simulink model "saved3"  (R2018b)
settings: Solver=VariableStepAuto  StartTime=0.0  StopTime=10.0  RelTol=1e-3
libraries: simulink x95, powerlib x8, powerlib_meascontrol x2
(part 3 of 6)

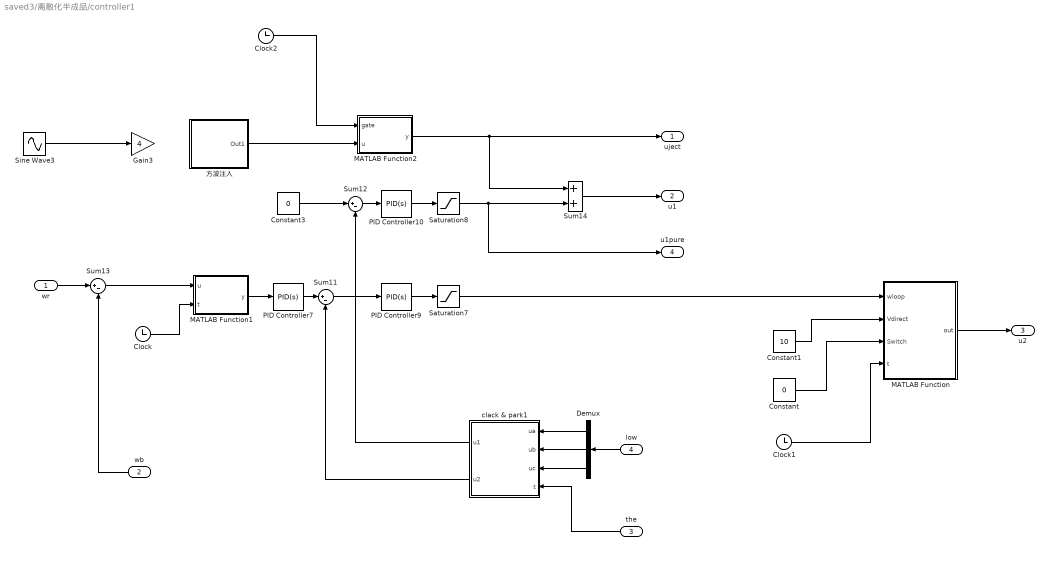
== system saved3/离散化半成品/controller1 ==
  wr : Inport
  wb : Inport  Port=2
  the : Inport  Port=3
  low : Inport  Port=4
  Clock : Clock
  Clock1 : Clock
  Clock2 : Clock
  Constant : Constant  Value=0
  Constant1 : Constant  Value=10
  Constant3 : Constant  Value=0
  Demux : Demux  Outputs=3
  Gain3 : Gain  Gain=4
  MATLAB Function : MATLAB Function  TreatAsAtomicUnit=on
  MATLAB Function1 : MATLAB Function  TreatAsAtomicUnit=on
  MATLAB Function2 : MATLAB Function  TreatAsAtomicUnit=on
  PID Controller10 : simulink/Continuous/PID Controller  Controller=PID  Form=Parallel  TimeDomain=Continuous-time  SampleTime=-1  IntegratorMethod=Forward Euler  FilterMethod=Forward Euler  ControllerParametersSource=internal  P=3  I=10  D=0  UseFilter=on  N=100  TunerSelectOption=Transfer Function Based (PID Tuner App)  InitialConditionSource=internal  InitialConditionForIntegrator=0  InitialConditionForFilter=0  DifferentiatorICPrevScaledInput=0  ExternalReset=none  TrackingMode=off  Kt=1  LimitOutput=off  UpperSaturationLimit=inf  LowerSaturationLimit=-inf  LinearizeAsGain=on  AntiWindupMode=none  Kb=1  POutMin=[]  POutMax=[]  IOutMin=[]  IOutMax=[]  DOutMin=[]  DOutMax=[]  NOutMin=[]  NOutMax=[]  SumOutMin=[]  SumOutMax=[]  SaturationOutMin=[]  SaturationOutMax=[]  PParamMin=[]  PParamMax=[]  IParamMin=[]  IParamMax=[]  DParamMin=[]  DParamMax=[]  NParamMin=[]  NParamMax=[]  KbParamMin=[]  KbParamMax=[]  KtParamMin=[]  KtParamMax=[]  KbOutMin=[]  KbOutMax=[]  KtOutMin=[]  KtOutMax=[]  IntegratorOutMin=[]  IntegratorOutMax=[]  FilterOutMin=[]  FilterOutMax=[]  SumI1OutMin=[]  SumI1OutMax=[]  SumI2OutMin=[]  SumI2OutMax=[]  SumI3OutMin=[]  SumI3OutMax=[]  SumI4OutMin=[]  SumI4OutMax=[]  SumDOutMin=[]  SumDOutMax=[]  DifferentiatorOutMin=[]  DifferentiatorOutMax=[]  FilterDiffOutCoefMin=[]  FilterDiffOutCoefMax=[]  ReciprocalOutMin=[]  ReciprocalOutMax=[]  SumDenOutMin=[]  SumDenOutMax=[]  SumNumOutMin=[]  SumNumOutMax=[]  DivideOutMin=[]  DivideOutMax=[]  IntegratorContinuousStateAttributes=''  IntegratorStateMustResolveToSignalObject=off  IntegratorRTWStateStorageClass=Auto  FilterContinuousStateAttributes=''  FilterStateMustResolveToSignalObject=off  FilterRTWStateStorageClass=Auto  ParallelPVariant=InternalParameters  IdealPVariant=Disabled  IVariant=InternalParameters  DVariant=InternalParameters  IntegratorVariant=Continuous  SatVariant=Disabled  AWVariant=Passthrough  PCopyVariant=Disabled  TRVariant=Disabled  FdbkBlocksVariant=Forward  IdealPFdbkVariant=Disabled  SatFdbkVariant=Disabled  DerivativeFilterVariant=ContFilter  NVariant=InternalParameters  NCopyVariant=Disabled  FilterICVariant=InternalICsFilter  IntegratorICVariant=InternalICs  ExternalResetVariant=Disabled  TRSumVariant=Passthrough  SumFdbkVariant=Disabled  SumVariant=Sum_PID
  PID Controller7 : simulink/Continuous/PID Controller  Controller=PID  Form=Parallel  TimeDomain=Continuous-time  SampleTime=1e-4  IntegratorMethod=Forward Euler  FilterMethod=Forward Euler  ControllerParametersSource=internal  P=0.3  I=5  D=0  UseFilter=on  N=100  TunerSelectOption=Transfer Function Based (PID Tuner App)  InitialConditionSource=internal  InitialConditionForIntegrator=0  InitialConditionForFilter=0  DifferentiatorICPrevScaledInput=0  ExternalReset=none  TrackingMode=off  Kt=1  LimitOutput=off  UpperSaturationLimit=inf  LowerSaturationLimit=-inf  LinearizeAsGain=on  AntiWindupMode=none  Kb=1  POutMin=[]  POutMax=[]  IOutMin=[]  IOutMax=[]  DOutMin=[]  DOutMax=[]  NOutMin=[]  NOutMax=[]  SumOutMin=[]  SumOutMax=[]  SaturationOutMin=[]  SaturationOutMax=[]  PParamMin=[]  PParamMax=[]  IParamMin=[]  IParamMax=[]  DParamMin=[]  DParamMax=[]  NParamMin=[]  NParamMax=[]  KbParamMin=[]  KbParamMax=[]  KtParamMin=[]  KtParamMax=[]  KbOutMin=[]  KbOutMax=[]  KtOutMin=[]  KtOutMax=[]  IntegratorOutMin=[]  IntegratorOutMax=[]  FilterOutMin=[]  FilterOutMax=[]  SumI1OutMin=[]  SumI1OutMax=[]  SumI2OutMin=[]  SumI2OutMax=[]  SumI3OutMin=[]  SumI3OutMax=[]  SumI4OutMin=[]  SumI4OutMax=[]  SumDOutMin=[]  SumDOutMax=[]  DifferentiatorOutMin=[]  DifferentiatorOutMax=[]  FilterDiffOutCoefMin=[]  FilterDiffOutCoefMax=[]  ReciprocalOutMin=[]  ReciprocalOutMax=[]  SumDenOutMin=[]  SumDenOutMax=[]  SumNumOutMin=[]  SumNumOutMax=[]  DivideOutMin=[]  DivideOutMax=[]  IntegratorContinuousStateAttributes=''  IntegratorStateMustResolveToSignalObject=off  IntegratorRTWStateStorageClass=Auto  FilterContinuousStateAttributes=''  FilterStateMustResolveToSignalObject=off  FilterRTWStateStorageClass=Auto  ParallelPVariant=InternalParameters  IdealPVariant=Disabled  IVariant=InternalParameters  DVariant=InternalParameters  IntegratorVariant=Continuous  SatVariant=Disabled  AWVariant=Passthrough  PCopyVariant=Disabled  TRVariant=Disabled  FdbkBlocksVariant=Forward  IdealPFdbkVariant=Disabled  SatFdbkVariant=Disabled  DerivativeFilterVariant=ContFilter  NVariant=InternalParameters  NCopyVariant=Disabled  FilterICVariant=InternalICsFilter  IntegratorICVariant=InternalICs  ExternalResetVariant=Disabled  TRSumVariant=Passthrough  SumFdbkVariant=Disabled  SumVariant=Sum_PID
  PID Controller9 : simulink/Continuous/PID Controller  Controller=PID  Form=Parallel  TimeDomain=Continuous-time  SampleTime=-1  IntegratorMethod=Forward Euler  FilterMethod=Forward Euler  ControllerParametersSource=internal  P=3  I=10  D=0  UseFilter=on  N=100  TunerSelectOption=Transfer Function Based (PID Tuner App)  InitialConditionSource=internal  InitialConditionForIntegrator=0  InitialConditionForFilter=0  DifferentiatorICPrevScaledInput=0  ExternalReset=none  TrackingMode=off  Kt=1  LimitOutput=off  UpperSaturationLimit=inf  LowerSaturationLimit=-inf  LinearizeAsGain=on  AntiWindupMode=none  Kb=1  POutMin=[]  POutMax=[]  IOutMin=[]  IOutMax=[]  DOutMin=[]  DOutMax=[]  NOutMin=[]  NOutMax=[]  SumOutMin=[]  SumOutMax=[]  SaturationOutMin=[]  SaturationOutMax=[]  PParamMin=[]  PParamMax=[]  IParamMin=[]  IParamMax=[]  DParamMin=[]  DParamMax=[]  NParamMin=[]  NParamMax=[]  KbParamMin=[]  KbParamMax=[]  KtParamMin=[]  KtParamMax=[]  KbOutMin=[]  KbOutMax=[]  KtOutMin=[]  KtOutMax=[]  IntegratorOutMin=[]  IntegratorOutMax=[]  FilterOutMin=[]  FilterOutMax=[]  SumI1OutMin=[]  SumI1OutMax=[]  SumI2OutMin=[]  SumI2OutMax=[]  SumI3OutMin=[]  SumI3OutMax=[]  SumI4OutMin=[]  SumI4OutMax=[]  SumDOutMin=[]  SumDOutMax=[]  DifferentiatorOutMin=[]  DifferentiatorOutMax=[]  FilterDiffOutCoefMin=[]  FilterDiffOutCoefMax=[]  ReciprocalOutMin=[]  ReciprocalOutMax=[]  SumDenOutMin=[]  SumDenOutMax=[]  SumNumOutMin=[]  SumNumOutMax=[]  DivideOutMin=[]  DivideOutMax=[]  IntegratorContinuousStateAttributes=''  IntegratorStateMustResolveToSignalObject=off  IntegratorRTWStateStorageClass=Auto  FilterContinuousStateAttributes=''  FilterStateMustResolveToSignalObject=off  FilterRTWStateStorageClass=Auto  ParallelPVariant=InternalParameters  IdealPVariant=Disabled  IVariant=InternalParameters  DVariant=InternalParameters  IntegratorVariant=Continuous  SatVariant=Disabled  AWVariant=Passthrough  PCopyVariant=Disabled  TRVariant=Disabled  FdbkBlocksVariant=Forward  IdealPFdbkVariant=Disabled  SatFdbkVariant=Disabled  DerivativeFilterVariant=ContFilter  NVariant=InternalParameters  NCopyVariant=Disabled  FilterICVariant=InternalICsFilter  IntegratorICVariant=InternalICs  ExternalResetVariant=Disabled  TRSumVariant=Passthrough  SumFdbkVariant=Disabled  SumVariant=Sum_PID
  Saturation7 : Saturate  UpperLimit=20  LowerLimit=-20
  Saturation8 : Saturate  UpperLimit=20  LowerLimit=-20
  Sine Wave3 : Sin  Frequency=1000*2*pi  SampleTime=0
  Sum11 : Sum  Inputs=|+-
  Sum12 : Sum  Inputs=|+-
  Sum13 : Sum  Inputs=|+-
  Sum14 : Sum
  clack & park1 : MATLAB Function  TreatAsAtomicUnit=on
  方波注入 : Subsystem
  uject : Outport
  u1 : Outport  Port=2
  u2 : Outport  Port=3
  u1pure : Outport  Port=4
  wires:
  Sum11/1 -> PID Controller9/1
  wb/1 -> Sum13/2
  Clock/1 -> MATLAB Function1/2(t)
  Saturation8/1 -> u1pure/1, Sum14/2
  MATLAB Function1/1(y) -> PID Controller7/1
  Sum13/1 -> MATLAB Function1/1(u)
  Constant3/1 -> Sum12/1
  PID Controller9/1 -> Saturation7/1
  Sum14/1 -> u1/1
  方波注入/1(Out1) -> MATLAB Function2/2(u)
  PID Controller7/1 -> Sum11/1
  Sum12/1 -> PID Controller10/1
  PID Controller10/1 -> Saturation8/1
  Sine Wave3/1 -> Gain3/1
  Saturation7/1 -> MATLAB Function/1(wloop)
  wr/1 -> Sum13/1
  MATLAB Function/1(out) -> u2/1
  Clock1/1 -> MATLAB Function/4(t)
  Constant/1 -> MATLAB Function/3(Switch)
  Constant1/1 -> MATLAB Function/2(Vdirect)
  Demux/1 -> clack & park1/1(ua)
  Demux/2 -> clack & park1/2(ub)
  Demux/3 -> clack & park1/3(uc)
  clack & park1/1(u1) -> Sum12/2
  clack & park1/2(u2) -> Sum11/2
  the/1 -> clack & park1/4(t)
  low/1 -> Demux/1
  MATLAB Function2/1(y) -> Sum14/1, uject/1
  Clock2/1 -> MATLAB Function2/1(gate)

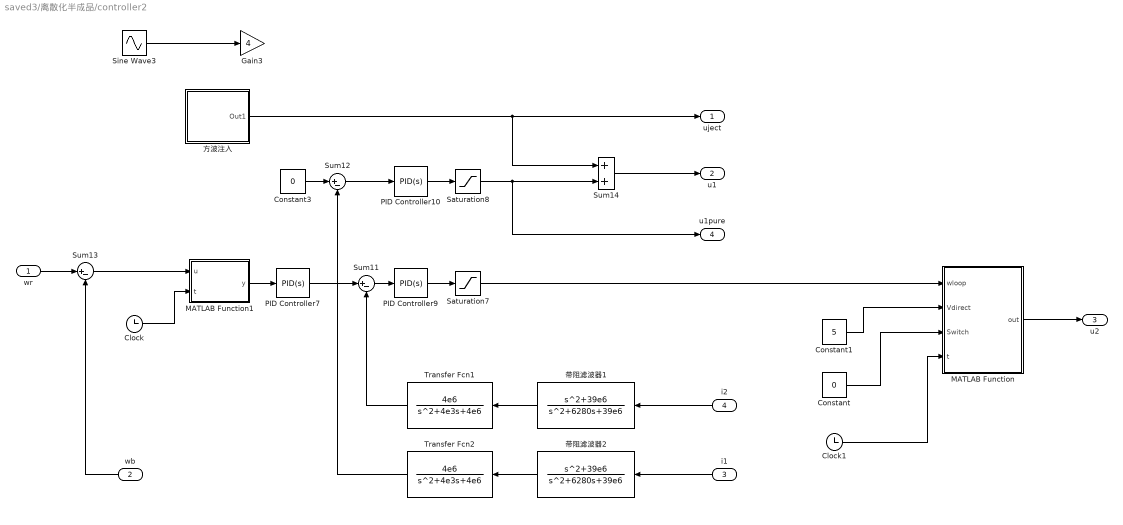
== system saved3/离散化半成品/controller2 ==
  wr : Inport
  wb : Inport  Port=2
  i1 : Inport  Port=3
  i2 : Inport  Port=4
  Clock : Clock
  Clock1 : Clock
  Constant : Constant  Value=0
  Constant1 : Constant  Value=5
  Constant3 : Constant  Value=0
  Gain3 : Gain  Gain=4
  MATLAB Function : MATLAB Function  TreatAsAtomicUnit=on
  MATLAB Function1 : MATLAB Function  TreatAsAtomicUnit=on
  PID Controller10 : simulink/Continuous/PID Controller  Controller=PID  Form=Parallel  TimeDomain=Continuous-time  SampleTime=-1  IntegratorMethod=Forward Euler  FilterMethod=Forward Euler  ControllerParametersSource=internal  P=3  I=10  D=0  UseFilter=on  N=100  TunerSelectOption=Transfer Function Based (PID Tuner App)  InitialConditionSource=internal  InitialConditionForIntegrator=0  InitialConditionForFilter=0  DifferentiatorICPrevScaledInput=0  ExternalReset=none  TrackingMode=off  Kt=1  LimitOutput=off  UpperSaturationLimit=inf  LowerSaturationLimit=-inf  LinearizeAsGain=on  AntiWindupMode=none  Kb=1  POutMin=[]  POutMax=[]  IOutMin=[]  IOutMax=[]  DOutMin=[]  DOutMax=[]  NOutMin=[]  NOutMax=[]  SumOutMin=[]  SumOutMax=[]  SaturationOutMin=[]  SaturationOutMax=[]  PParamMin=[]  PParamMax=[]  IParamMin=[]  IParamMax=[]  DParamMin=[]  DParamMax=[]  NParamMin=[]  NParamMax=[]  KbParamMin=[]  KbParamMax=[]  KtParamMin=[]  KtParamMax=[]  KbOutMin=[]  KbOutMax=[]  KtOutMin=[]  KtOutMax=[]  IntegratorOutMin=[]  IntegratorOutMax=[]  FilterOutMin=[]  FilterOutMax=[]  SumI1OutMin=[]  SumI1OutMax=[]  SumI2OutMin=[]  SumI2OutMax=[]  SumI3OutMin=[]  SumI3OutMax=[]  SumI4OutMin=[]  SumI4OutMax=[]  SumDOutMin=[]  SumDOutMax=[]  DifferentiatorOutMin=[]  DifferentiatorOutMax=[]  FilterDiffOutCoefMin=[]  FilterDiffOutCoefMax=[]  ReciprocalOutMin=[]  ReciprocalOutMax=[]  SumDenOutMin=[]  SumDenOutMax=[]  SumNumOutMin=[]  SumNumOutMax=[]  DivideOutMin=[]  DivideOutMax=[]  IntegratorContinuousStateAttributes=''  IntegratorStateMustResolveToSignalObject=off  IntegratorRTWStateStorageClass=Auto  FilterContinuousStateAttributes=''  FilterStateMustResolveToSignalObject=off  FilterRTWStateStorageClass=Auto  ParallelPVariant=InternalParameters  IdealPVariant=Disabled  IVariant=InternalParameters  DVariant=InternalParameters  IntegratorVariant=Continuous  SatVariant=Disabled  AWVariant=Passthrough  PCopyVariant=Disabled  TRVariant=Disabled  FdbkBlocksVariant=Forward  IdealPFdbkVariant=Disabled  SatFdbkVariant=Disabled  DerivativeFilterVariant=ContFilter  NVariant=InternalParameters  NCopyVariant=Disabled  FilterICVariant=InternalICsFilter  IntegratorICVariant=InternalICs  ExternalResetVariant=Disabled  TRSumVariant=Passthrough  SumFdbkVariant=Disabled  SumVariant=Sum_PID
  PID Controller7 : simulink/Continuous/PID Controller  Controller=PID  Form=Parallel  TimeDomain=Continuous-time  SampleTime=1e-4  IntegratorMethod=Forward Euler  FilterMethod=Forward Euler  ControllerParametersSource=internal  P=0.3  I=5  D=0  UseFilter=on  N=100  TunerSelectOption=Transfer Function Based (PID Tuner App)  InitialConditionSource=internal  InitialConditionForIntegrator=0  InitialConditionForFilter=0  DifferentiatorICPrevScaledInput=0  ExternalReset=none  TrackingMode=off  Kt=1  LimitOutput=off  UpperSaturationLimit=inf  LowerSaturationLimit=-inf  LinearizeAsGain=on  AntiWindupMode=none  Kb=1  POutMin=[]  POutMax=[]  IOutMin=[]  IOutMax=[]  DOutMin=[]  DOutMax=[]  NOutMin=[]  NOutMax=[]  SumOutMin=[]  SumOutMax=[]  SaturationOutMin=[]  SaturationOutMax=[]  PParamMin=[]  PParamMax=[]  IParamMin=[]  IParamMax=[]  DParamMin=[]  DParamMax=[]  NParamMin=[]  NParamMax=[]  KbParamMin=[]  KbParamMax=[]  KtParamMin=[]  KtParamMax=[]  KbOutMin=[]  KbOutMax=[]  KtOutMin=[]  KtOutMax=[]  IntegratorOutMin=[]  IntegratorOutMax=[]  FilterOutMin=[]  FilterOutMax=[]  SumI1OutMin=[]  SumI1OutMax=[]  SumI2OutMin=[]  SumI2OutMax=[]  SumI3OutMin=[]  SumI3OutMax=[]  SumI4OutMin=[]  SumI4OutMax=[]  SumDOutMin=[]  SumDOutMax=[]  DifferentiatorOutMin=[]  DifferentiatorOutMax=[]  FilterDiffOutCoefMin=[]  FilterDiffOutCoefMax=[]  ReciprocalOutMin=[]  ReciprocalOutMax=[]  SumDenOutMin=[]  SumDenOutMax=[]  SumNumOutMin=[]  SumNumOutMax=[]  DivideOutMin=[]  DivideOutMax=[]  IntegratorContinuousStateAttributes=''  IntegratorStateMustResolveToSignalObject=off  IntegratorRTWStateStorageClass=Auto  FilterContinuousStateAttributes=''  FilterStateMustResolveToSignalObject=off  FilterRTWStateStorageClass=Auto  ParallelPVariant=InternalParameters  IdealPVariant=Disabled  IVariant=InternalParameters  DVariant=InternalParameters  IntegratorVariant=Continuous  SatVariant=Disabled  AWVariant=Passthrough  PCopyVariant=Disabled  TRVariant=Disabled  FdbkBlocksVariant=Forward  IdealPFdbkVariant=Disabled  SatFdbkVariant=Disabled  DerivativeFilterVariant=ContFilter  NVariant=InternalParameters  NCopyVariant=Disabled  FilterICVariant=InternalICsFilter  IntegratorICVariant=InternalICs  ExternalResetVariant=Disabled  TRSumVariant=Passthrough  SumFdbkVariant=Disabled  SumVariant=Sum_PID
  PID Controller9 : simulink/Continuous/PID Controller  Controller=PID  Form=Parallel  TimeDomain=Continuous-time  SampleTime=-1  IntegratorMethod=Forward Euler  FilterMethod=Forward Euler  ControllerParametersSource=internal  P=3  I=10  D=0  UseFilter=on  N=100  TunerSelectOption=Transfer Function Based (PID Tuner App)  InitialConditionSource=internal  InitialConditionForIntegrator=0  InitialConditionForFilter=0  DifferentiatorICPrevScaledInput=0  ExternalReset=none  TrackingMode=off  Kt=1  LimitOutput=off  UpperSaturationLimit=inf  LowerSaturationLimit=-inf  LinearizeAsGain=on  AntiWindupMode=none  Kb=1  POutMin=[]  POutMax=[]  IOutMin=[]  IOutMax=[]  DOutMin=[]  DOutMax=[]  NOutMin=[]  NOutMax=[]  SumOutMin=[]  SumOutMax=[]  SaturationOutMin=[]  SaturationOutMax=[]  PParamMin=[]  PParamMax=[]  IParamMin=[]  IParamMax=[]  DParamMin=[]  DParamMax=[]  NParamMin=[]  NParamMax=[]  KbParamMin=[]  KbParamMax=[]  KtParamMin=[]  KtParamMax=[]  KbOutMin=[]  KbOutMax=[]  KtOutMin=[]  KtOutMax=[]  IntegratorOutMin=[]  IntegratorOutMax=[]  FilterOutMin=[]  FilterOutMax=[]  SumI1OutMin=[]  SumI1OutMax=[]  SumI2OutMin=[]  SumI2OutMax=[]  SumI3OutMin=[]  SumI3OutMax=[]  SumI4OutMin=[]  SumI4OutMax=[]  SumDOutMin=[]  SumDOutMax=[]  DifferentiatorOutMin=[]  DifferentiatorOutMax=[]  FilterDiffOutCoefMin=[]  FilterDiffOutCoefMax=[]  ReciprocalOutMin=[]  ReciprocalOutMax=[]  SumDenOutMin=[]  SumDenOutMax=[]  SumNumOutMin=[]  SumNumOutMax=[]  DivideOutMin=[]  DivideOutMax=[]  IntegratorContinuousStateAttributes=''  IntegratorStateMustResolveToSignalObject=off  IntegratorRTWStateStorageClass=Auto  FilterContinuousStateAttributes=''  FilterStateMustResolveToSignalObject=off  FilterRTWStateStorageClass=Auto  ParallelPVariant=InternalParameters  IdealPVariant=Disabled  IVariant=InternalParameters  DVariant=InternalParameters  IntegratorVariant=Continuous  SatVariant=Disabled  AWVariant=Passthrough  PCopyVariant=Disabled  TRVariant=Disabled  FdbkBlocksVariant=Forward  IdealPFdbkVariant=Disabled  SatFdbkVariant=Disabled  DerivativeFilterVariant=ContFilter  NVariant=InternalParameters  NCopyVariant=Disabled  FilterICVariant=InternalICsFilter  IntegratorICVariant=InternalICs  ExternalResetVariant=Disabled  TRSumVariant=Passthrough  SumFdbkVariant=Disabled  SumVariant=Sum_PID
  Saturation7 : Saturate  UpperLimit=20  LowerLimit=-20
  Saturation8 : Saturate  UpperLimit=20  LowerLimit=-20
  Sine Wave3 : Sin  Frequency=1000*2*pi  SampleTime=0
  Sum11 : Sum  Inputs=|+-
  Sum12 : Sum  Inputs=|+-
  Sum13 : Sum  Inputs=|+-
  Sum14 : Sum
  Transfer Fcn1 : TransferFcn  Numerator=[4e6]  Denominator=[1 4e3 4e6]
  Transfer Fcn2 : TransferFcn  Numerator=[4e6]  Denominator=[1 4e3 4e6]
  带阻滤波器1 : TransferFcn  Numerator=[1 0 39e6]  Denominator=[1 6280 39e6]
  带阻滤波器2 : TransferFcn  Numerator=[1 0 39e6]  Denominator=[1 6280 39e6]
  方波注入 : Subsystem
  uject : Outport
  u1 : Outport  Port=2
  u2 : Outport  Port=3
  u1pure : Outport  Port=4
  wires:
  Sum11/1 -> PID Controller9/1
  wb/1 -> Sum13/2
  Clock/1 -> MATLAB Function1/2(t)
  Saturation8/1 -> u1pure/1, Sum14/2
  MATLAB Function1/1(y) -> PID Controller7/1
  Sum13/1 -> MATLAB Function1/1(u)
  Constant3/1 -> Sum12/1
  PID Controller9/1 -> Saturation7/1
  Sum14/1 -> u1/1
  方波注入/1(Out1) -> uject/1, Sum14/1
  PID Controller7/1 -> Sum11/1
  Sum12/1 -> PID Controller10/1
  PID Controller10/1 -> Saturation8/1
  Sine Wave3/1 -> Gain3/1
  i2/1 -> 带阻滤波器1/1
  带阻滤波器2/1 -> Transfer Fcn2/1
  带阻滤波器1/1 -> Transfer Fcn1/1
  i1/1 -> 带阻滤波器2/1
  Saturation7/1 -> MATLAB Function/1(wloop)
  wr/1 -> Sum13/1
  Transfer Fcn1/1 -> Sum11/2
  Transfer Fcn2/1 -> Sum12/2
  MATLAB Function/1(out) -> u2/1
  Clock1/1 -> MATLAB Function/4(t)
  Constant/1 -> MATLAB Function/3(Switch)
  Constant1/1 -> MATLAB Function/2(Vdirect)

== system saved3/离散化半成品/controller3 ==
  wr : Inport
  wb : Inport  Port=2
  i1 : Inport  Port=3
  i2 : Inport  Port=4
  Clock : Clock
  Clock1 : Clock
  Constant : Constant
  Constant1 : Constant  Value=10
  Constant3 : Constant  Value=0
  Gain3 : Gain  Gain=4
  MATLAB Function : MATLAB Function  TreatAsAtomicUnit=on
  MATLAB Function1 : MATLAB Function  TreatAsAtomicUnit=on
  PID Controller10 : simulink/Continuous/PID Controller  Controller=PID  Form=Parallel  TimeDomain=Continuous-time  SampleTime=-1  IntegratorMethod=Forward Euler  FilterMethod=Forward Euler  ControllerParametersSource=internal  P=3  I=10  D=0  UseFilter=on  N=100  TunerSelectOption=Transfer Function Based (PID Tuner App)  InitialConditionSource=internal  InitialConditionForIntegrator=0  InitialConditionForFilter=0  DifferentiatorICPrevScaledInput=0  ExternalReset=none  TrackingMode=off  Kt=1  LimitOutput=off  UpperSaturationLimit=inf  LowerSaturationLimit=-inf  LinearizeAsGain=on  AntiWindupMode=none  Kb=1  POutMin=[]  POutMax=[]  IOutMin=[]  IOutMax=[]  DOutMin=[]  DOutMax=[]  NOutMin=[]  NOutMax=[]  SumOutMin=[]  SumOutMax=[]  SaturationOutMin=[]  SaturationOutMax=[]  PParamMin=[]  PParamMax=[]  IParamMin=[]  IParamMax=[]  DParamMin=[]  DParamMax=[]  NParamMin=[]  NParamMax=[]  KbParamMin=[]  KbParamMax=[]  KtParamMin=[]  KtParamMax=[]  KbOutMin=[]  KbOutMax=[]  KtOutMin=[]  KtOutMax=[]  IntegratorOutMin=[]  IntegratorOutMax=[]  FilterOutMin=[]  FilterOutMax=[]  SumI1OutMin=[]  SumI1OutMax=[]  SumI2OutMin=[]  SumI2OutMax=[]  SumI3OutMin=[]  SumI3OutMax=[]  SumI4OutMin=[]  SumI4OutMax=[]  SumDOutMin=[]  SumDOutMax=[]  DifferentiatorOutMin=[]  DifferentiatorOutMax=[]  FilterDiffOutCoefMin=[]  FilterDiffOutCoefMax=[]  ReciprocalOutMin=[]  ReciprocalOutMax=[]  SumDenOutMin=[]  SumDenOutMax=[]  SumNumOutMin=[]  SumNumOutMax=[]  DivideOutMin=[]  DivideOutMax=[]  IntegratorContinuousStateAttributes=''  IntegratorStateMustResolveToSignalObject=off  IntegratorRTWStateStorageClass=Auto  FilterContinuousStateAttributes=''  FilterStateMustResolveToSignalObject=off  FilterRTWStateStorageClass=Auto  ParallelPVariant=InternalParameters  IdealPVariant=Disabled  IVariant=InternalParameters  DVariant=InternalParameters  IntegratorVariant=Continuous  SatVariant=Disabled  AWVariant=Passthrough  PCopyVariant=Disabled  TRVariant=Disabled  FdbkBlocksVariant=Forward  IdealPFdbkVariant=Disabled  SatFdbkVariant=Disabled  DerivativeFilterVariant=ContFilter  NVariant=InternalParameters  NCopyVariant=Disabled  FilterICVariant=InternalICsFilter  IntegratorICVariant=InternalICs  ExternalResetVariant=Disabled  TRSumVariant=Passthrough  SumFdbkVariant=Disabled  SumVariant=Sum_PID
  PID Controller7 : simulink/Continuous/PID Controller  Controller=PID  Form=Parallel  TimeDomain=Continuous-time  SampleTime=1e-4  IntegratorMethod=Forward Euler  FilterMethod=Forward Euler  ControllerParametersSource=internal  P=0.3  I=5  D=0  UseFilter=on  N=100  TunerSelectOption=Transfer Function Based (PID Tuner App)  InitialConditionSource=internal  InitialConditionForIntegrator=0  InitialConditionForFilter=0  DifferentiatorICPrevScaledInput=0  ExternalReset=none  TrackingMode=off  Kt=1  LimitOutput=off  UpperSaturationLimit=inf  LowerSaturationLimit=-inf  LinearizeAsGain=on  AntiWindupMode=none  Kb=1  POutMin=[]  POutMax=[]  IOutMin=[]  IOutMax=[]  DOutMin=[]  DOutMax=[]  NOutMin=[]  NOutMax=[]  SumOutMin=[]  SumOutMax=[]  SaturationOutMin=[]  SaturationOutMax=[]  PParamMin=[]  PParamMax=[]  IParamMin=[]  IParamMax=[]  DParamMin=[]  DParamMax=[]  NParamMin=[]  NParamMax=[]  KbParamMin=[]  KbParamMax=[]  KtParamMin=[]  KtParamMax=[]  KbOutMin=[]  KbOutMax=[]  KtOutMin=[]  KtOutMax=[]  IntegratorOutMin=[]  IntegratorOutMax=[]  FilterOutMin=[]  FilterOutMax=[]  SumI1OutMin=[]  SumI1OutMax=[]  SumI2OutMin=[]  SumI2OutMax=[]  SumI3OutMin=[]  SumI3OutMax=[]  SumI4OutMin=[]  SumI4OutMax=[]  SumDOutMin=[]  SumDOutMax=[]  DifferentiatorOutMin=[]  DifferentiatorOutMax=[]  FilterDiffOutCoefMin=[]  FilterDiffOutCoefMax=[]  ReciprocalOutMin=[]  ReciprocalOutMax=[]  SumDenOutMin=[]  SumDenOutMax=[]  SumNumOutMin=[]  SumNumOutMax=[]  DivideOutMin=[]  DivideOutMax=[]  IntegratorContinuousStateAttributes=''  IntegratorStateMustResolveToSignalObject=off  IntegratorRTWStateStorageClass=Auto  FilterContinuousStateAttributes=''  FilterStateMustResolveToSignalObject=off  FilterRTWStateStorageClass=Auto  ParallelPVariant=InternalParameters  IdealPVariant=Disabled  IVariant=InternalParameters  DVariant=InternalParameters  IntegratorVariant=Continuous  SatVariant=Disabled  AWVariant=Passthrough  PCopyVariant=Disabled  TRVariant=Disabled  FdbkBlocksVariant=Forward  IdealPFdbkVariant=Disabled  SatFdbkVariant=Disabled  DerivativeFilterVariant=ContFilter  NVariant=InternalParameters  NCopyVariant=Disabled  FilterICVariant=InternalICsFilter  IntegratorICVariant=InternalICs  ExternalResetVariant=Disabled  TRSumVariant=Passthrough  SumFdbkVariant=Disabled  SumVariant=Sum_PID
  PID Controller9 : simulink/Continuous/PID Controller  Controller=PID  Form=Parallel  TimeDomain=Continuous-time  SampleTime=-1  IntegratorMethod=Forward Euler  FilterMethod=Forward Euler  ControllerParametersSource=internal  P=3  I=10  D=0  UseFilter=on  N=100  TunerSelectOption=Transfer Function Based (PID Tuner App)  InitialConditionSource=internal  InitialConditionForIntegrator=0  InitialConditionForFilter=0  DifferentiatorICPrevScaledInput=0  ExternalReset=none  TrackingMode=off  Kt=1  LimitOutput=off  UpperSaturationLimit=inf  LowerSaturationLimit=-inf  LinearizeAsGain=on  AntiWindupMode=none  Kb=1  POutMin=[]  POutMax=[]  IOutMin=[]  IOutMax=[]  DOutMin=[]  DOutMax=[]  NOutMin=[]  NOutMax=[]  SumOutMin=[]  SumOutMax=[]  SaturationOutMin=[]  SaturationOutMax=[]  PParamMin=[]  PParamMax=[]  IParamMin=[]  IParamMax=[]  DParamMin=[]  DParamMax=[]  NParamMin=[]  NParamMax=[]  KbParamMin=[]  KbParamMax=[]  KtParamMin=[]  KtParamMax=[]  KbOutMin=[]  KbOutMax=[]  KtOutMin=[]  KtOutMax=[]  IntegratorOutMin=[]  IntegratorOutMax=[]  FilterOutMin=[]  FilterOutMax=[]  SumI1OutMin=[]  SumI1OutMax=[]  SumI2OutMin=[]  SumI2OutMax=[]  SumI3OutMin=[]  SumI3OutMax=[]  SumI4OutMin=[]  SumI4OutMax=[]  SumDOutMin=[]  SumDOutMax=[]  DifferentiatorOutMin=[]  DifferentiatorOutMax=[]  FilterDiffOutCoefMin=[]  FilterDiffOutCoefMax=[]  ReciprocalOutMin=[]  ReciprocalOutMax=[]  SumDenOutMin=[]  SumDenOutMax=[]  SumNumOutMin=[]  SumNumOutMax=[]  DivideOutMin=[]  DivideOutMax=[]  IntegratorContinuousStateAttributes=''  IntegratorStateMustResolveToSignalObject=off  IntegratorRTWStateStorageClass=Auto  FilterContinuousStateAttributes=''  FilterStateMustResolveToSignalObject=off  FilterRTWStateStorageClass=Auto  ParallelPVariant=InternalParameters  IdealPVariant=Disabled  IVariant=InternalParameters  DVariant=InternalParameters  IntegratorVariant=Continuous  SatVariant=Disabled  AWVariant=Passthrough  PCopyVariant=Disabled  TRVariant=Disabled  FdbkBlocksVariant=Forward  IdealPFdbkVariant=Disabled  SatFdbkVariant=Disabled  DerivativeFilterVariant=ContFilter  NVariant=InternalParameters  NCopyVariant=Disabled  FilterICVariant=InternalICsFilter  IntegratorICVariant=InternalICs  ExternalResetVariant=Disabled  TRSumVariant=Passthrough  SumFdbkVariant=Disabled  SumVariant=Sum_PID
  Saturation7 : Saturate  UpperLimit=20  LowerLimit=-20
  Saturation8 : Saturate  UpperLimit=20  LowerLimit=-20
  Sine Wave3 : Sin  Frequency=1000*2*pi  SampleTime=0
  Sum11 : Sum  Inputs=|+-
  Sum12 : Sum  Inputs=|+-
  Sum13 : Sum  Inputs=|+-
  Sum14 : Sum
  Transfer Fcn1 : TransferFcn  Numerator=[4e6]  Denominator=[1 4e3 4e6]
  Transfer Fcn2 : TransferFcn  Numerator=[4e6]  Denominator=[1 4e3 4e6]
  带阻滤波器1 : TransferFcn  Numerator=[1 0 39e6]  Denominator=[1 6280 39e6]
  带阻滤波器2 : TransferFcn  Numerator=[1 0 39e6]  Denominator=[1 6280 39e6]
  方波注入 : Subsystem
  uject : Outport
  u1 : Outport  Port=2
  u2 : Outport  Port=3
  u1pure : Outport  Port=4
  wires:
  Sum11/1 -> PID Controller9/1
  wb/1 -> Sum13/2
  Clock/1 -> MATLAB Function1/2(t)
  Saturation8/1 -> u1pure/1, Sum14/2
  MATLAB Function1/1(y) -> PID Controller7/1
  Sum13/1 -> MATLAB Function1/1(u)
  Constant3/1 -> Sum12/1
  PID Controller9/1 -> Saturation7/1
  Sum14/1 -> u1/1
  方波注入/1(Out1) -> uject/1, Sum14/1
  PID Controller7/1 -> Sum11/1
  Sum12/1 -> PID Controller10/1
  PID Controller10/1 -> Saturation8/1
  Sine Wave3/1 -> Gain3/1
  i2/1 -> 带阻滤波器1/1
  带阻滤波器2/1 -> Transfer Fcn2/1
  带阻滤波器1/1 -> Transfer Fcn1/1
  i1/1 -> 带阻滤波器2/1
  Saturation7/1 -> MATLAB Function/1(wloop)
  wr/1 -> Sum13/1
  Transfer Fcn1/1 -> Sum11/2
  Transfer Fcn2/1 -> Sum12/2
  MATLAB Function/1(out) -> u2/1
  Clock1/1 -> MATLAB Function/4(t)
  Constant/1 -> MATLAB Function/3(Switch)
  Constant1/1 -> MATLAB Function/2(Vdirect)

== system saved3/离散化半成品/current seperator ==
  ia : Inport
  ib : Inport  Port=2
  ic : Inport  Port=3
  Mux : Mux  Inputs=3
  Mux1 : Mux  Inputs=3
  Transfer Fcn : TransferFcn  Numerator=[4e6]  Denominator=[1 4e3 4e6]
  Transfer Fcn1 : TransferFcn  Numerator=[6280 0]  Denominator=[1 6280 39e6]
  Transfer Fcn2 : TransferFcn  Numerator=[4e6]  Denominator=[1 4e3 4e6]
  Transfer Fcn3 : TransferFcn  Numerator=[6280 0]  Denominator=[1 6280 39e6]
  Transfer Fcn4 : TransferFcn  Numerator=[6280 0]  Denominator=[1 6280 39e6]
  Transfer Fcn5 : TransferFcn  Numerator=[4e6]  Denominator=[1 4e3 4e6]
  带通滤波器1 : TransferFcn  Numerator=[6280 0]  Denominator=[1 6280 39e6]
  带通滤波器3 : TransferFcn  Numerator=[6280 0]  Denominator=[1 6280 39e6]
  带通滤波器4 : TransferFcn  Numerator=[6280 0]  Denominator=[1 6280 39e6]
  带阻滤波器 : TransferFcn  Numerator=[1 0 39e6]  Denominator=[1 6280 39e6]
  带阻滤波器1 : TransferFcn  Numerator=[1 0 39e6]  Denominator=[1 6280 39e6]
  带阻滤波器2 : TransferFcn  Numerator=[1 0 39e6]  Denominator=[1 6280 39e6]
  电流采样 : Subsystem
  电流采样1 : Subsystem
  1000Hz : Outport
  low : Outport  Port=2
  wires:
  Mux/1 -> 1000Hz/1
  带通滤波器3/1 -> Transfer Fcn3/1
  Transfer Fcn1/1 -> 电流采样/1(<Stator current is_a (A)>)
  电流采样/2(ib) -> Mux/2
  电流采样/3(ic) -> Mux/3
  电流采样/1(ia) -> Mux/1
  Transfer Fcn3/1 -> 电流采样/2(<Stator current is_b (A)>)
  Transfer Fcn4/1 -> 电流采样/3(<Stator current is_c (A)>)
  带通滤波器1/1 -> Transfer Fcn1/1
  带通滤波器4/1 -> Transfer Fcn4/1
  ia/1 -> 带阻滤波器1/1, 带通滤波器1/1
  ib/1 -> 带阻滤波器/1, 带通滤波器3/1
  ic/1 -> 带阻滤波器2/1, 带通滤波器4/1
  带阻滤波器1/1 -> Transfer Fcn/1
  带阻滤波器/1 -> Transfer Fcn2/1
  Transfer Fcn2/1 -> 电流采样1/2(<Stator current is_b (A)>)
  Transfer Fcn/1 -> 电流采样1/1(<Stator current is_a (A)>)
  Transfer Fcn5/1 -> 电流采样1/3(<Stator current is_c (A)>)
  Mux1/1 -> low/1
  电流采样1/1(ia) -> Mux1/1
  电流采样1/2(ib) -> Mux1/2
  电流采样1/3(ic) -> Mux1/3
  带阻滤波器2/1 -> Transfer Fcn5/1

== system saved3/离散化半成品/inject estimater ==
  uject : Inport
  u2 : Inport  Port=2
  Gain6 : Gain  Gain=0.01
  Gain8 : Gain  Gain=-100
  Integrator2 : Integrator  InitialCondition=0.3
  PID Controller2 : simulink/Continuous/PID Controller  Controller=PID  Form=Parallel  TimeDomain=Continuous-time  SampleTime=-1  IntegratorMethod=Forward Euler  FilterMethod=Forward Euler  ControllerParametersSource=internal  P=4  I=350  D=0  UseFilter=on  N=100  TunerSelectOption=Transfer Function Based (PID Tuner App)  InitialConditionSource=internal  InitialConditionForIntegrator=0  InitialConditionForFilter=0  DifferentiatorICPrevScaledInput=0  ExternalReset=none  TrackingMode=off  Kt=1  LimitOutput=off  UpperSaturationLimit=inf  LowerSaturationLimit=-inf  LinearizeAsGain=on  AntiWindupMode=none  Kb=1  POutMin=[]  POutMax=[]  IOutMin=[]  IOutMax=[]  DOutMin=[]  DOutMax=[]  NOutMin=[]  NOutMax=[]  SumOutMin=[]  SumOutMax=[]  SaturationOutMin=[]  SaturationOutMax=[]  PParamMin=[]  PParamMax=[]  IParamMin=[]  IParamMax=[]  DParamMin=[]  DParamMax=[]  NParamMin=[]  NParamMax=[]  KbParamMin=[]  KbParamMax=[]  KtParamMin=[]  KtParamMax=[]  KbOutMin=[]  KbOutMax=[]  KtOutMin=[]  KtOutMax=[]  IntegratorOutMin=[]  IntegratorOutMax=[]  FilterOutMin=[]  FilterOutMax=[]  SumI1OutMin=[]  SumI1OutMax=[]  SumI2OutMin=[]  SumI2OutMax=[]  SumI3OutMin=[]  SumI3OutMax=[]  SumI4OutMin=[]  SumI4OutMax=[]  SumDOutMin=[]  SumDOutMax=[]  DifferentiatorOutMin=[]  DifferentiatorOutMax=[]  FilterDiffOutCoefMin=[]  FilterDiffOutCoefMax=[]  ReciprocalOutMin=[]  ReciprocalOutMax=[]  SumDenOutMin=[]  SumDenOutMax=[]  SumNumOutMin=[]  SumNumOutMax=[]  DivideOutMin=[]  DivideOutMax=[]  IntegratorContinuousStateAttributes=''  IntegratorStateMustResolveToSignalObject=off  IntegratorRTWStateStorageClass=Auto  FilterContinuousStateAttributes=''  FilterStateMustResolveToSignalObject=off  FilterRTWStateStorageClass=Auto  ParallelPVariant=InternalParameters  IdealPVariant=Disabled  IVariant=InternalParameters  DVariant=InternalParameters  IntegratorVariant=Continuous  SatVariant=Disabled  AWVariant=Passthrough  PCopyVariant=Disabled  TRVariant=Disabled  FdbkBlocksVariant=Forward  IdealPFdbkVariant=Disabled  SatFdbkVariant=Disabled  DerivativeFilterVariant=ContFilter  NVariant=InternalParameters  NCopyVariant=Disabled  FilterICVariant=InternalICsFilter  IntegratorICVariant=InternalICs  ExternalResetVariant=Disabled  TRSumVariant=Passthrough  SumFdbkVariant=Disabled  SumVariant=Sum_PID
  Ramp2 : simulink/Sources/Ramp  slope=0  start=0  InitialOutput=0
  Scope19 : Scope
  Scope7 : Scope  NumInputPorts=2
  Sum2 : Sum  Inputs=|++
  Transfer Fcn2 : TransferFcn  Numerator=[6280 0]  Denominator=[1 6280 39e6]
  低通滤波器 : TransferFcn  Numerator=[25e4]  Denominator=[1 500 25e4]
  带通滤波器1 : TransferFcn  Numerator=[6280 0]  Denominator=[1 6280 39e6]
  带通滤波器2 : TransferFcn  Numerator=[6280 0]  Denominator=[1 6280 39e6]
  混频 : Product
  相移器-90° : TransferFcn  Numerator=[39e6]  Denominator=[1 6280 39e6]
  theHat : Outport
  wHat : Outport  Port=2
  wires:
  相移器-90°/1 -> 混频/1
  混频/1 -> 低通滤波器/1
  Gain6/1 -> Scope7/1
  带通滤波器2/1 -> Transfer Fcn2/1
  Transfer Fcn2/1 -> 相移器-90°/1, Scope7/2
  PID Controller2/1 -> Sum2/1
  Integrator2/1 -> theHat/1
  Gain8/1 -> PID Controller2/1
  Ramp2/1 -> Sum2/2
  带通滤波器1/1 -> 混频/2, Gain6/1
  u2/1 -> 带通滤波器2/1
  uject/1 -> 带通滤波器1/1
  Sum2/1 -> wHat/1, Integrator2/1
  低通滤波器/1 -> Gain8/1, Scope19/1

== system saved3/离散化半成品/inject estimater(digital) ==
  uject : Inport
  u2 : Inport  Port=2
  Constant : Constant  Value=1000
  Constant1 : Constant  Value=0.3
  Gain1 : Gain  Gain=-3
  Gain6 : Gain  Gain=0.01
  Scope : Scope
  Scope1 : Scope  NumInputPorts=2
  Sum : Sum  Inputs=|++
  Transfer Fcn2 : TransferFcn  Numerator=[6280 0]  Denominator=[1 6280 39e6]
  乘法 : Product
  带通滤波器2 : TransferFcn  Numerator=[6280 0]  Denominator=[1 6280 39e6]
  鉴幅鉴相器(可选快速门滑窗) : MATLAB Function  TreatAsAtomicUnit=on  SystemSampleTime=1e-4
  锁相器 : MATLAB Function  TreatAsAtomicUnit=on  SystemSampleTime=1e-4
  theHat : Outport
  wHat : Outport  Port=2
  wires:
  带通滤波器2/1 -> Transfer Fcn2/1
  Transfer Fcn2/1 -> 鉴幅鉴相器(可选快速门滑窗)/2(S2), Scope1/2
  Gain1/1 -> 锁相器/1(u)
  uject/1 -> 鉴幅鉴相器(可选快速门滑窗)/1(S1), Gain6/1
  u2/1 -> 带通滤波器2/1
  鉴幅鉴相器(可选快速门滑窗)/2(A2) -> 乘法/1
  鉴幅鉴相器(可选快速门滑窗)/3(DP) -> 乘法/2  "phase"
  乘法/1 -> Gain1/1, Scope/1
  Constant/1 -> 鉴幅鉴相器(可选快速门滑窗)/3(Fre)
  Gain6/1 -> Scope1/1
  Sum/1 -> theHat/1
  Constant1/1 -> Sum/2
  锁相器/1(the) -> Sum/1
  锁相器/2(w) -> wHat/1

== system saved3/离散化半成品/inject estimater(digital)1 ==
  uject : Inport
  In3 : Inport  Port=2
  Constant2 : Constant  Value=1000
  Constant3 : Constant  Value=0.3
  Delay : Delay  DelayLength=1
  Demux : Demux  Outputs=3
  Gain2 : Gain  Gain=-3
  Gain3 : Gain  Gain=0.01
  Scope2 : Scope
  Scope3 : Scope  NumInputPorts=2
  Sum1 : Sum  Inputs=|++
  clack & park2 : MATLAB Function  TreatAsAtomicUnit=on
  乘法1 : Product
  鉴幅鉴相器(可选快速门滑窗)1 : MATLAB Function  TreatAsAtomicUnit=on  SystemSampleTime=1e-4
  锁相器1 : MATLAB Function  TreatAsAtomicUnit=on  SystemSampleTime=1e-4
  the : Outport
  wHat : Outport  Port=2
  wires:
  uject/1 -> 鉴幅鉴相器(可选快速门滑窗)1/1(S1), Gain3/1
  In3/1 -> Demux/1
  Gain2/1 -> 锁相器1/1(u)
  Constant2/1 -> 鉴幅鉴相器(可选快速门滑窗)1/3(Fre)
  鉴幅鉴相器(可选快速门滑窗)1/3(DP) -> 乘法1/2  "phase"
  鉴幅鉴相器(可选快速门滑窗)1/2(A2) -> 乘法1/1
  乘法1/1 -> Gain2/1, Scope2/1
  Gain3/1 -> Scope3/1
  Constant3/1 -> Sum1/2
  Demux/1 -> clack & park2/1(ua)
  Demux/2 -> clack & park2/2(ub)
  Demux/3 -> clack & park2/3(uc)
  锁相器1/2(w) -> wHat/1
  锁相器1/1(the) -> Sum1/1
  Sum1/1 -> Delay/1, the/1
  clack & park2/2(u2) -> 鉴幅鉴相器(可选快速门滑窗)1/2(S2), Scope3/2
  Delay/1 -> clack & park2/4(t)

== system saved3/离散化半成品/inject estimater(digital)2 ==
  uject : Inport
  In3 : Inport  Port=2
  Constant2 : Constant  Value=1000
  Constant3 : Constant  Value=0.3
  Delay : Delay  DelayLength=1
  Demux : Demux  Outputs=3
  Gain2 : Gain  Gain=-3
  Gain3 : Gain  Gain=0.01
  Scope2 : Scope
  Scope3 : Scope  NumInputPorts=2
  Sum1 : Sum  Inputs=|++
  clack & park2 : MATLAB Function  TreatAsAtomicUnit=on
  乘法1 : Product
  鉴幅鉴相器(可选快速门滑窗)1 : MATLAB Function  TreatAsAtomicUnit=on  SystemSampleTime=1e-4
  锁相器1 : MATLAB Function  TreatAsAtomicUnit=on  SystemSampleTime=1e-4
  the : Outport
  wHat : Outport  Port=2
  wires:
  uject/1 -> 鉴幅鉴相器(可选快速门滑窗)1/1(S1), Gain3/1
  In3/1 -> Demux/1
  Gain2/1 -> 锁相器1/1(u)
  Constant2/1 -> 鉴幅鉴相器(可选快速门滑窗)1/3(Fre)
  鉴幅鉴相器(可选快速门滑窗)1/3(DP) -> 乘法1/2  "phase"
  鉴幅鉴相器(可选快速门滑窗)1/2(A2) -> 乘法1/1
  乘法1/1 -> Gain2/1, Scope2/1
  Gain3/1 -> Scope3/1
  Constant3/1 -> Sum1/2
  Demux/1 -> clack & park2/1(ua)
  Demux/2 -> clack & park2/2(ub)
  Demux/3 -> clack & park2/3(uc)
  锁相器1/2(w) -> wHat/1
  锁相器1/1(the) -> Sum1/1
  Sum1/1 -> Delay/1, the/1
  clack & park2/2(u2) -> 鉴幅鉴相器(可选快速门滑窗)1/2(S2), Scope3/2
  Delay/1 -> clack & park2/4(t)

== system saved3/离散化半成品/inject estimater(digital)3 ==
  uject : Inport
  u2 : Inport  Port=2
  Constant : Constant  Value=1000
  Constant1 : Constant  Value=0.3
  Gain1 : Gain  Gain=-3
  Gain6 : Gain  Gain=0.01
  Scope : Scope
  Scope1 : Scope  NumInputPorts=2
  Sum : Sum  Inputs=|++
  Transfer Fcn2 : TransferFcn  Numerator=[6280 0]  Denominator=[1 6280 39e6]
  乘法 : Product
  带通滤波器2 : TransferFcn  Numerator=[6280 0]  Denominator=[1 6280 39e6]
  鉴幅鉴相器(可选快速门滑窗) : MATLAB Function  TreatAsAtomicUnit=on  SystemSampleTime=1e-4
  锁相器 : MATLAB Function  TreatAsAtomicUnit=on  SystemSampleTime=1e-4
  theHat : Outport
  wHat : Outport  Port=2
  wires:
  带通滤波器2/1 -> Transfer Fcn2/1
  Transfer Fcn2/1 -> 鉴幅鉴相器(可选快速门滑窗)/2(S2), Scope1/2
  Gain1/1 -> 锁相器/1(u)
  uject/1 -> 鉴幅鉴相器(可选快速门滑窗)/1(S1), Gain6/1
  u2/1 -> 带通滤波器2/1
  鉴幅鉴相器(可选快速门滑窗)/2(A2) -> 乘法/1
  鉴幅鉴相器(可选快速门滑窗)/3(DP) -> 乘法/2  "phase"
  乘法/1 -> Gain1/1, Scope/1
  Constant/1 -> 鉴幅鉴相器(可选快速门滑窗)/3(Fre)
  Gain6/1 -> Scope1/1
  Sum/1 -> theHat/1
  Constant1/1 -> Sum/2
  锁相器/1(the) -> Sum/1
  锁相器/2(w) -> wHat/1

== system saved3/离散化半成品/inject estimater1 ==
  uject : Inport
  u2 : Inport  Port=2
  Gain6 : Gain  Gain=0.01
  Gain8 : Gain  Gain=-100
  Integrator2 : Integrator  InitialCondition=0.3
  PID Controller2 : simulink/Continuous/PID Controller  Controller=PID  Form=Parallel  TimeDomain=Continuous-time  SampleTime=-1  IntegratorMethod=Forward Euler  FilterMethod=Forward Euler  ControllerParametersSource=internal  P=4  I=350  D=0  UseFilter=on  N=100  TunerSelectOption=Transfer Function Based (PID Tuner App)  InitialConditionSource=internal  InitialConditionForIntegrator=0  InitialConditionForFilter=0  DifferentiatorICPrevScaledInput=0  ExternalReset=none  TrackingMode=off  Kt=1  LimitOutput=off  UpperSaturationLimit=inf  LowerSaturationLimit=-inf  LinearizeAsGain=on  AntiWindupMode=none  Kb=1  POutMin=[]  POutMax=[]  IOutMin=[]  IOutMax=[]  DOutMin=[]  DOutMax=[]  NOutMin=[]  NOutMax=[]  SumOutMin=[]  SumOutMax=[]  SaturationOutMin=[]  SaturationOutMax=[]  PParamMin=[]  PParamMax=[]  IParamMin=[]  IParamMax=[]  DParamMin=[]  DParamMax=[]  NParamMin=[]  NParamMax=[]  KbParamMin=[]  KbParamMax=[]  KtParamMin=[]  KtParamMax=[]  KbOutMin=[]  KbOutMax=[]  KtOutMin=[]  KtOutMax=[]  IntegratorOutMin=[]  IntegratorOutMax=[]  FilterOutMin=[]  FilterOutMax=[]  SumI1OutMin=[]  SumI1OutMax=[]  SumI2OutMin=[]  SumI2OutMax=[]  SumI3OutMin=[]  SumI3OutMax=[]  SumI4OutMin=[]  SumI4OutMax=[]  SumDOutMin=[]  SumDOutMax=[]  DifferentiatorOutMin=[]  DifferentiatorOutMax=[]  FilterDiffOutCoefMin=[]  FilterDiffOutCoefMax=[]  ReciprocalOutMin=[]  ReciprocalOutMax=[]  SumDenOutMin=[]  SumDenOutMax=[]  SumNumOutMin=[]  SumNumOutMax=[]  DivideOutMin=[]  DivideOutMax=[]  IntegratorContinuousStateAttributes=''  IntegratorStateMustResolveToSignalObject=off  IntegratorRTWStateStorageClass=Auto  FilterContinuousStateAttributes=''  FilterStateMustResolveToSignalObject=off  FilterRTWStateStorageClass=Auto  ParallelPVariant=InternalParameters  IdealPVariant=Disabled  IVariant=InternalParameters  DVariant=InternalParameters  IntegratorVariant=Continuous  SatVariant=Disabled  AWVariant=Passthrough  PCopyVariant=Disabled  TRVariant=Disabled  FdbkBlocksVariant=Forward  IdealPFdbkVariant=Disabled  SatFdbkVariant=Disabled  DerivativeFilterVariant=ContFilter  NVariant=InternalParameters  NCopyVariant=Disabled  FilterICVariant=InternalICsFilter  IntegratorICVariant=InternalICs  ExternalResetVariant=Disabled  TRSumVariant=Passthrough  SumFdbkVariant=Disabled  SumVariant=Sum_PID
  Ramp2 : simulink/Sources/Ramp  slope=0  start=0  InitialOutput=0
  Scope19 : Scope
  Scope7 : Scope  NumInputPorts=2
  Sum2 : Sum  Inputs=|++
  Transfer Fcn2 : TransferFcn  Numerator=[6280 0]  Denominator=[1 6280 39e6]
  低通滤波器 : TransferFcn  Numerator=[25e4]  Denominator=[1 500 25e4]
  带通滤波器1 : TransferFcn  Numerator=[6280 0]  Denominator=[1 6280 39e6]
  带通滤波器2 : TransferFcn  Numerator=[6280 0]  Denominator=[1 6280 39e6]
  混频 : Product
  相移器-90° : TransferFcn  Numerator=[39e6]  Denominator=[1 6280 39e6]
  theHat : Outport
  wHat : Outport  Port=2
  wires:
  相移器-90°/1 -> 混频/1
  混频/1 -> 低通滤波器/1
  Gain6/1 -> Scope7/1
  带通滤波器2/1 -> Transfer Fcn2/1
  Transfer Fcn2/1 -> 相移器-90°/1, Scope7/2
  PID Controller2/1 -> Sum2/1
  Integrator2/1 -> theHat/1
  Gain8/1 -> PID Controller2/1
  Ramp2/1 -> Sum2/2
  带通滤波器1/1 -> 混频/2, Gain6/1
  u2/1 -> 带通滤波器2/1
  uject/1 -> 带通滤波器1/1
  Sum2/1 -> wHat/1, Integrator2/1
  低通滤波器/1 -> Gain8/1, Scope19/1

== system saved3/离散化半成品/inject estimater2 ==
  uject : Inport
  u2 : Inport  Port=2
  Gain6 : Gain  Gain=0.01
  Gain8 : Gain  Gain=-100
  Integrator2 : Integrator  InitialCondition=0.3
  PID Controller2 : simulink/Continuous/PID Controller  Controller=PID  Form=Parallel  TimeDomain=Continuous-time  SampleTime=-1  IntegratorMethod=Forward Euler  FilterMethod=Forward Euler  ControllerParametersSource=internal  P=4  I=350  D=0  UseFilter=on  N=100  TunerSelectOption=Transfer Function Based (PID Tuner App)  InitialConditionSource=internal  InitialConditionForIntegrator=0  InitialConditionForFilter=0  DifferentiatorICPrevScaledInput=0  ExternalReset=none  TrackingMode=off  Kt=1  LimitOutput=off  UpperSaturationLimit=inf  LowerSaturationLimit=-inf  LinearizeAsGain=on  AntiWindupMode=none  Kb=1  POutMin=[]  POutMax=[]  IOutMin=[]  IOutMax=[]  DOutMin=[]  DOutMax=[]  NOutMin=[]  NOutMax=[]  SumOutMin=[]  SumOutMax=[]  SaturationOutMin=[]  SaturationOutMax=[]  PParamMin=[]  PParamMax=[]  IParamMin=[]  IParamMax=[]  DParamMin=[]  DParamMax=[]  NParamMin=[]  NParamMax=[]  KbParamMin=[]  KbParamMax=[]  KtParamMin=[]  KtParamMax=[]  KbOutMin=[]  KbOutMax=[]  KtOutMin=[]  KtOutMax=[]  IntegratorOutMin=[]  IntegratorOutMax=[]  FilterOutMin=[]  FilterOutMax=[]  SumI1OutMin=[]  SumI1OutMax=[]  SumI2OutMin=[]  SumI2OutMax=[]  SumI3OutMin=[]  SumI3OutMax=[]  SumI4OutMin=[]  SumI4OutMax=[]  SumDOutMin=[]  SumDOutMax=[]  DifferentiatorOutMin=[]  DifferentiatorOutMax=[]  FilterDiffOutCoefMin=[]  FilterDiffOutCoefMax=[]  ReciprocalOutMin=[]  ReciprocalOutMax=[]  SumDenOutMin=[]  SumDenOutMax=[]  SumNumOutMin=[]  SumNumOutMax=[]  DivideOutMin=[]  DivideOutMax=[]  IntegratorContinuousStateAttributes=''  IntegratorStateMustResolveToSignalObject=off  IntegratorRTWStateStorageClass=Auto  FilterContinuousStateAttributes=''  FilterStateMustResolveToSignalObject=off  FilterRTWStateStorageClass=Auto  ParallelPVariant=InternalParameters  IdealPVariant=Disabled  IVariant=InternalParameters  DVariant=InternalParameters  IntegratorVariant=Continuous  SatVariant=Disabled  AWVariant=Passthrough  PCopyVariant=Disabled  TRVariant=Disabled  FdbkBlocksVariant=Forward  IdealPFdbkVariant=Disabled  SatFdbkVariant=Disabled  DerivativeFilterVariant=ContFilter  NVariant=InternalParameters  NCopyVariant=Disabled  FilterICVariant=InternalICsFilter  IntegratorICVariant=InternalICs  ExternalResetVariant=Disabled  TRSumVariant=Passthrough  SumFdbkVariant=Disabled  SumVariant=Sum_PID
  Ramp2 : simulink/Sources/Ramp  slope=0  start=0  InitialOutput=0
  Scope19 : Scope
  Scope7 : Scope  NumInputPorts=2
  Sum2 : Sum  Inputs=|++
  Transfer Fcn2 : TransferFcn  Numerator=[6280 0]  Denominator=[1 6280 39e6]
  低通滤波器 : TransferFcn  Numerator=[25e4]  Denominator=[1 500 25e4]
  带通滤波器1 : TransferFcn  Numerator=[6280 0]  Denominator=[1 6280 39e6]
  带通滤波器2 : TransferFcn  Numerator=[6280 0]  Denominator=[1 6280 39e6]
  混频 : Product
  相移器-90° : TransferFcn  Numerator=[39e6]  Denominator=[1 6280 39e6]
  theHat : Outport
  wHat : Outport  Port=2
  wires:
  相移器-90°/1 -> 混频/1
  混频/1 -> 低通滤波器/1
  Gain6/1 -> Scope7/1
  带通滤波器2/1 -> Transfer Fcn2/1
  Transfer Fcn2/1 -> 相移器-90°/1, Scope7/2
  PID Controller2/1 -> Sum2/1
  Integrator2/1 -> theHat/1
  Gain8/1 -> PID Controller2/1
  Ramp2/1 -> Sum2/2
  带通滤波器1/1 -> 混频/2, Gain6/1
  u2/1 -> 带通滤波器2/1
  uject/1 -> 带通滤波器1/1
  Sum2/1 -> wHat/1, Integrator2/1
  低通滤波器/1 -> Gain8/1, Scope19/1

== system saved3/离散化半成品/w estimater ==
  u1pure : Inport
  u2 : Inport  Port=2
  ia : Inport  Port=3
  ib : Inport  Port=4
  ic : Inport  Port=5
  the : Inport  Port=6
  MATLAB Function : MATLAB Function  TreatAsAtomicUnit=on
  Subsystem : Subsystem
  Transfer Fcn : TransferFcn  Numerator=[4e6]  Denominator=[1 4e3 4e6]
  Transfer Fcn1 : TransferFcn  Numerator=[4e6]  Denominator=[1 4e3 4e6]
  clack : MATLAB Function  TreatAsAtomicUnit=on
  iabc : Scope  NumInputPorts=3
  invpark : MATLAB Function  TreatAsAtomicUnit=on
  带阻滤波器 : TransferFcn  Numerator=[1 0 39e6]  Denominator=[1 6280 39e6]
  带阻滤波器1 : TransferFcn  Numerator=[1 0 39e6]  Denominator=[1 6280 39e6]
  锁相环 : Subsystem
  wHat : Outport
  theHat : Outport  Port=2
  wires:
  ib/1 -> clack/2(ib), iabc/2
  Subsystem/1(Ea) -> MATLAB Function/1(Ea), 锁相环/1(cos)
  Subsystem/2(Eb) -> MATLAB Function/2(Eb), 锁相环/2(sin)
  invpark/2(ub) -> Subsystem/2(ub)
  clack/1(iap) -> 带阻滤波器/1
  u2/1 -> invpark/2(u2)
  clack/2(ibe) -> 带阻滤波器1/1
  invpark/1(ua) -> Subsystem/1(ua)
  ia/1 -> clack/1(ia), iabc/1
  ic/1 -> clack/3(ic), iabc/3
  u1pure/1 -> invpark/1(u1)
  the/1 -> invpark/3(t)
  锁相环/1(we) -> wHat/1
  带阻滤波器1/1 -> Transfer Fcn/1
  带阻滤波器/1 -> Transfer Fcn1/1
  Transfer Fcn1/1 -> Subsystem/3(ia)
  Transfer Fcn/1 -> Subsystem/4(ib)
  MATLAB Function/1(y) -> theHat/1

== system saved3/离散化半成品/w estimater1 ==
  u1pure : Inport
  u2 : Inport  Port=2
  low : Inport  Port=3
  the : Inport  Port=4
  Delay : Delay  DelayLength=1
  Demux : Demux  Outputs=3
  Mux : Mux
  Subsystem1 : Subsystem
  clack1 : MATLAB Function  TreatAsAtomicUnit=on
  invpark : MATLAB Function  TreatAsAtomicUnit=on
  磁链观测器 : MATLAB Function  TreatAsAtomicUnit=on  SystemSampleTime=1e-4
  锁相环1 : Subsystem
  wHat : Outport
  theHat : Outport  Port=2
  wires:
  invpark/2(ub) -> Mux/2, Subsystem1/2(ub)
  u2/1 -> invpark/2(u2)
  invpark/1(ua) -> Mux/1, Subsystem1/1(ua)
  u1pure/1 -> invpark/1(u1)
  the/1 -> invpark/3(t)
  Demux/1 -> clack1/1(ia)
  Demux/2 -> clack1/2(ib)
  Demux/3 -> clack1/3(ic)
  Subsystem1/1(Ea) -> 锁相环1/1(cos)
  Subsystem1/2(Eb) -> 锁相环1/2(sin)
  clack1/1(iap) -> Mux/3, Subsystem1/3(ia)
  clack1/2(ibe) -> Mux/4, Subsystem1/4(ib)
  low/1 -> Demux/1
  锁相环1/1(we) -> wHat/1
  磁链观测器/1(y) -> Delay/1
  Mux/1 -> 磁链观测器/1(u)
  Delay/1 -> theHat/1

== system saved3/离散化半成品/w estimater2 ==
  u1pure : Inport
  u2 : Inport  Port=2
  ia : Inport  Port=3
  ib : Inport  Port=4
  ic : Inport  Port=5
  the : Inport  Port=6
  MATLAB Function : MATLAB Function  TreatAsAtomicUnit=on
  Subsystem : Subsystem
  Transfer Fcn : TransferFcn  Numerator=[4e6]  Denominator=[1 4e3 4e6]
  Transfer Fcn1 : TransferFcn  Numerator=[4e6]  Denominator=[1 4e3 4e6]
  clack : MATLAB Function  TreatAsAtomicUnit=on
  iabc : Scope  NumInputPorts=3
  invpark : MATLAB Function  TreatAsAtomicUnit=on
  带阻滤波器 : TransferFcn  Numerator=[1 0 39e6]  Denominator=[1 6280 39e6]
  带阻滤波器1 : TransferFcn  Numerator=[1 0 39e6]  Denominator=[1 6280 39e6]
  锁相环 : Subsystem
  wHat : Outport
  theHat : Outport  Port=2
  wires:
  ib/1 -> clack/2(ib), iabc/2
  Subsystem/1(Ea) -> MATLAB Function/1(Ea), 锁相环/1(cos)
  Subsystem/2(Eb) -> MATLAB Function/2(Eb), 锁相环/2(sin)
  invpark/2(ub) -> Subsystem/2(ub)
  clack/1(iap) -> 带阻滤波器/1
  u2/1 -> invpark/2(u2)
  clack/2(ibe) -> 带阻滤波器1/1
  invpark/1(ua) -> Subsystem/1(ua)
  ia/1 -> clack/1(ia), iabc/1
  ic/1 -> clack/3(ic), iabc/3
  u1pure/1 -> invpark/1(u1)
  the/1 -> invpark/3(t)
  锁相环/1(we) -> wHat/1
  带阻滤波器1/1 -> Transfer Fcn/1
  带阻滤波器/1 -> Transfer Fcn1/1
  Transfer Fcn1/1 -> Subsystem/3(ia)
  Transfer Fcn/1 -> Subsystem/4(ib)
  MATLAB Function/1(y) -> theHat/1

== system saved3/离散化半成品/w estimater3 ==
  u1pure : Inport
  u2 : Inport  Port=2
  ia : Inport  Port=3
  ib : Inport  Port=4
  ic : Inport  Port=5
  the : Inport  Port=6
  Delay : Delay  DelayLength=1
  MATLAB Function : MATLAB Function  TreatAsAtomicUnit=on
  Mux : Mux
  Scope : Scope
  Subsystem : Subsystem
  Transfer Fcn : TransferFcn  Numerator=[4e6]  Denominator=[1 4e3 4e6]
  Transfer Fcn1 : TransferFcn  Numerator=[4e6]  Denominator=[1 4e3 4e6]
  clack : MATLAB Function  TreatAsAtomicUnit=on
  iabc : Scope  NumInputPorts=3
  invpark : MATLAB Function  TreatAsAtomicUnit=on
  带阻滤波器 : TransferFcn  Numerator=[1 0 39e6]  Denominator=[1 6280 39e6]
  带阻滤波器1 : TransferFcn  Numerator=[1 0 39e6]  Denominator=[1 6280 39e6]
  磁链观测器 : MATLAB Function  TreatAsAtomicUnit=on  SystemSampleTime=1e-4
  锁相环 : Subsystem
  wHat : Outport
  theHat : Outport  Port=2
  wires:
  ib/1 -> clack/2(ib), iabc/2
  Subsystem/1(Ea) -> MATLAB Function/1(Ea), 锁相环/1(cos)
  Subsystem/2(Eb) -> MATLAB Function/2(Eb), 锁相环/2(sin)
  invpark/2(ub) -> Subsystem/2(ub), Mux/2
  u2/1 -> invpark/2(u2)
  clack/2(ibe) -> 带阻滤波器1/1
  invpark/1(ua) -> Subsystem/1(ua), Mux/1
  ia/1 -> clack/1(ia), iabc/1
  ic/1 -> clack/3(ic), iabc/3
  u1pure/1 -> invpark/1(u1)
  the/1 -> invpark/3(t)
  锁相环/1(we) -> wHat/1
  带阻滤波器1/1 -> Transfer Fcn/1
  带阻滤波器/1 -> Transfer Fcn1/1
  Transfer Fcn1/1 -> Mux/3, Subsystem/3(ia)
  Transfer Fcn/1 -> Mux/4, Subsystem/4(ib)
  Mux/1 -> 磁链观测器/1(u)
  clack/1(iap) -> 带阻滤波器/1
  磁链观测器/1(y) -> Delay/1, Scope/1
  Delay/1 -> theHat/1

== system saved3/离散化半成品/电流采样 ==
  <Stator current is_a (A)> : Inport
  <Stator current is_b (A)> : Inport  Port=2
  <Stator current is_c (A)> : Inport  Port=3
  A/D转换 10KHz2 : MATLAB Function  TreatAsAtomicUnit=on  SystemSampleTime=1e-4
  A/D转换 10KHz3 : MATLAB Function  TreatAsAtomicUnit=on  SystemSampleTime=1e-4
  A/D转换 10KHz4 : MATLAB Function  TreatAsAtomicUnit=on  SystemSampleTime=1e-4
  Scope : Scope  NumInputPorts=3
  Sum1 : Sum  Inputs=|++
  Sum2 : Sum  Inputs=|++
  Sum3 : Sum  Inputs=|+-
  一阶滤波器40kHz1 : MATLAB Function  Commented=on  TreatAsAtomicUnit=on  SystemSampleTime=2.5e-5
  一阶滤波器40kHz2 : MATLAB Function  Commented=on  TreatAsAtomicUnit=on  SystemSampleTime=2.5e-5
  一阶滤波器40kHz3 : MATLAB Function  Commented=on  TreatAsAtomicUnit=on  SystemSampleTime=2.5e-5
  噪声 ia : simulink/Sources/Band-Limited White Noise  Cov=1e-7  Ts=1e-4  seed=[1]
  噪声 ib : simulink/Sources/Band-Limited White Noise  Cov=1e-7  Ts=1e-4  seed=[2]
  噪声 ic : simulink/Sources/Band-Limited White Noise  Cov=1e-7  Ts=1e-4  seed=[3]
  ia : Outport
  ib : Outport  Port=2
  ic : Outport  Port=3
  wires:
  Sum1/1 -> A/D转换 10KHz2/1(u)
  Sum2/1 -> A/D转换 10KHz3/1(u)
  Sum3/1 -> A/D转换 10KHz4/1(u)
  <Stator current is_b (A)>/1 -> Sum2/1
  <Stator current is_c (A)>/1 -> Sum3/1
  <Stator current is_a (A)>/1 -> Sum1/1
  A/D转换 10KHz2/1(y) -> Scope/1, ia/1
  A/D转换 10KHz3/1(y) -> Scope/2, ib/1
  A/D转换 10KHz4/1(y) -> Scope/3, ic/1
  噪声 ia/1 -> Sum1/2
  噪声 ib/1 -> Sum2/2
  噪声 ic/1 -> Sum3/2
